simulink model "Part3_simulazione"  (R2024b)
settings: Solver=ode4  StartTime=0.0  StopTime=T_SIM  FixedStep=T_s  RelTol=1e-3
values from neighbouring files (symbols this model uses):
  D = diag([0.001, 0.001, 0.0175/6, 0.0175/6, 0.0175/6, 0.0175/6*T_s, 0.0175/6*T_s].^2)    [P2_script.m]    (also in P3_script_usare_dati_veri.m; Parte2_corretto.m)
  d = 0.165    [P1_script.m]    (also in P1_script_vers2.m; P2_script.m; P3_script.m; P3_script_usare_dati_veri.m = 0.18428)
  d_id = d_cal_hat    [P2_script.m]    (also in P3_script_usare_dati_veri.m = 0.18428; Parte2_corretto.m)
  H_enc = [0, 0, 0, 1, 0, 0, 0 ... (first row only)    [P2_script.m]    (also in P3_script_usare_dati_veri.m; Parte2_corretto.m)
  H_gyro = [0, 0, 0, 0, 0, -r_id/d_id, r_id/d_id]    [P2_script.m]    (also in P3_script_usare_dati_veri.m; Parte2_corretto.m)
  H_motion_cap = [1, 0, 0, 0, 0, 0, 0 ... (first row only)    [P2_script.m]    (also in P3_script_usare_dati_veri.m; Parte2_corretto.m)
  omega_max = 10    [P1_script.m]    (also in P1_script_vers2.m; P2_script.m; P3_script.m; P3_script_usare_dati_veri.m)
  P_INIT_EKF = diag([0.001, 0.001, 0.0175/6, 0.0175/6, 0.0175/6, 0.0175/6*T_s, 0.0175/6*T_s].^2)    [P2_script.m]    (also in P3_script_usare_dati_veri.m; Parte2_corretto.m)
  p_loss = p_loss_values(3)    [P2_script.m]    (also in P3_script_usare_dati_veri.m = p_loss_values(i); Parte2_corretto.m = p_loss_values(2))
  PHI_INIT = [0;0]    [P1_script.m]    (also in P1_script_vers2.m; P2_script.m; P3_script_usare_dati_veri.m; Parte2_corretto.m)
  Q_INIT = [0; 0; atan2((R*omega_trj), (2*R*omega_trj))]    [P1_script.m]    (also in P1_script_vers2.m = q(:,1); P2_script.m = q_motion_capture_cal(1,:)'; P3_script_usare_dati_veri.m = q_motion_capture(1,:)'; Parte2_corretto.m = q_motion_capture_cal(1,:)')
  Q_INIT_LOC = Q_INIT    [P1_script.m]    (also in P1_script_vers2.m; P2_script.m; P3_script_usare_dati_veri.m = Q_INIT + [0.2; 0.2; deg2rad(15)]; Parte2_corretto.m)
  r = 0.03    [P1_script.m]    (also in P1_script_vers2.m; P2_script.m; P3_script.m; P3_script_usare_dati_veri.m = 0.03316)
  R_3 = diag(([var_motion_capture, var_motion_capture, var_motion_capture,               ENCODER_QUANTIZATION/6, ENCODER_QUANTIZATION/6, var_IMU]).^2)    [P2_script.m]    (also in P3_script_usare_dati_veri.m; Parte2_corretto.m)
  r_id = r_cal_hat    [P2_script.m]    (also in P3_script_usare_dati_veri.m = 0.03316; Parte2_corretto.m)
  T_s = 0.04    [P1_script.m]    (also in P1_script_vers2.m; P2_script.m; P3_script.m; P3_script_usare_dati_veri.m)
  Ts = 1e-2    (= 0.01)    [collaudo.m]
  Z_INIT_EKF = [Q_INIT; 0; 0; 0; 0]    [P1_script.m]    (also in P1_script_vers2.m; P2_script.m; P3_script_usare_dati_veri.m = [Q_INIT_LOC; 0; 0; 0; 0]; Parte2_corretto.m = [Q_INIT_LOC; 0; 0; 0; 0])
undefined symbols (not defined in the file or in its folder): X, Y
libraries: robotlib x5
settings Model: Creator=tomailoren  LastModifiedBy=loren
settings OptimizationCC: DefaultParameterBehavior=Inlined  EnhancedBackFolding=on  PassReuseOutputArgsAs=Individual arguments  ZeroExternalMemoryAtStartup=off  ZeroInternalMemoryAtStartup=off  MaxStackSize=64  OptimizeBlockOrder=speed  DifferentSizesBufferReuse=on  OptimizationCustomize=off  EfficientTunableParamExpr=on
settings DebuggingCC: ParameterTunabilityLossMsg=error
settings HardwareCC: ProdBitPerPointer=32  ProdBitPerSizeT=32  ProdBitPerPtrDiffT=32  ProdLargestAtomicFloat=None  ProdIntDivRoundTo=Undefined  ProdEndianess=Unspecified  ProdWordSize=32  ProdHWDeviceType=Generic->Unspecified (assume 32-bit Generic)
settings SFSimCC: MATLABDynamicMemAlloc=off
settings RTWCC: Description=Embedded Coder  SystemTargetFile=ert.tlc  HardwareBoard=Robot Operating System (ROS)  TLCOptions="-aInlineSetEventsForThisBaseRateFcn=TLC_FALSE -aSuppressMultiTaskScheduler=TLC_FALSE  -aRateBasedStepFcn=0"  TemplateMakefile=ert_default_tmf  Toolchain=Catkin  TargetLang=C++
settings CodeAppCC: ForceParamTrailComments=on  IgnoreCustomStorageClasses=off  OperatorAnnotations=on  SimulinkDataObjDesc=on  SFDataObjDesc=on  InsertBlockDesc=on

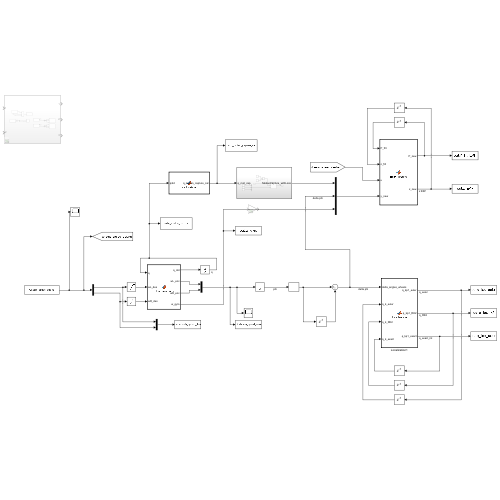
[thumbnail: Simulink's stored preview of the top-level diagram]
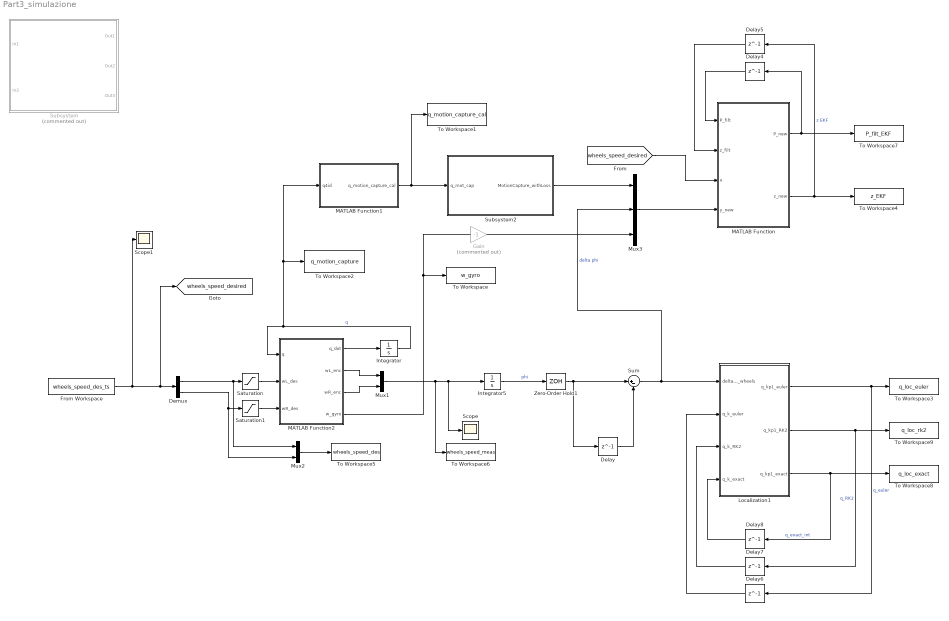
== system Part3_simulazione ==
  Delay : Delay  DelayLength=1  InitialCondition=[0;0]  SampleTime=T_s
  Delay4 : Delay  DelayLength=1  InitialCondition=P_INIT_EKF  SampleTime=T_s
  Delay5 : Delay  DelayLength=1  InitialCondition=Z_INIT_EKF  SampleTime=T_s
  Delay6 : Delay  DelayLength=1  InitialCondition=Q_INIT_LOC
  Delay7 : Delay  DelayLength=1  InitialCondition=Q_INIT_LOC
  Delay8 : Delay  DelayLength=1  InitialCondition=Q_INIT_LOC
  Demux : Demux  Outputs=2
  From Workspace : FromWorkspace  VariableName=wheels_speed_des_ts
  Gain : Gain  Commented=on  Gain=-1
  Integrator : Integrator  InitialCondition=Q_INIT
  Integrator5 : Integrator  InitialCondition=PHI_INIT
  Localization1 : MATLAB Function  TreatAsAtomicUnit=on
  MATLAB Function : MATLAB Function  TreatAsAtomicUnit=on
  MATLAB Function1 : MATLAB Function  TreatAsAtomicUnit=on
  MATLAB Function2 : MATLAB Function  TreatAsAtomicUnit=on
  Mux1 : Mux  Inputs=2
  Mux2 : Mux  Inputs=2
  Mux3 : Mux  Inputs=3
  Saturation : Saturate  UpperLimit=omega_max  LowerLimit=-omega_max
  Saturation1 : Saturate  UpperLimit=omega_max  LowerLimit=-omega_max
  Scope : Scope
  Scope1 : Scope
  Subsystem : Subsystem  Commented=on
  Subsystem2 : Subsystem
  Sum : Sum  Inputs=|+-
  To Workspace : ToWorkspace  VariableName=w_gyro  SaveFormat=Structure With Time  SampleTime=-1
  To Workspace1 : ToWorkspace  VariableName=q_motion_capture_cal  SaveFormat=Structure With Time  SampleTime=-1
  To Workspace2 : ToWorkspace  VariableName=q_motion_capture  SaveFormat=Structure With Time  SampleTime=-1
  To Workspace3 : ToWorkspace  VariableName=q_loc_euler  SaveFormat=Structure With Time  SampleTime=-1
  To Workspace4 : ToWorkspace  VariableName=z_EKF  SaveFormat=Structure With Time  SampleTime=-1
  To Workspace5 : ToWorkspace  VariableName=wheels_speed_des  SaveFormat=Structure With Time  SampleTime=-1
  To Workspace6 : ToWorkspace  VariableName=wheels_speed_meas  SaveFormat=Structure With Time  SampleTime=-1
  To Workspace7 : ToWorkspace  VariableName=P_filt_EKF  SaveFormat=Structure With Time  SampleTime=-1
  To Workspace8 : ToWorkspace  VariableName=q_loc_exact  SaveFormat=Structure With Time  SampleTime=-1
  To Workspace9 : ToWorkspace  VariableName=q_loc_rk2  SaveFormat=Structure With Time  SampleTime=-1
  Zero-Order Hold1 : ZeroOrderHold  SampleTime=T_s
  tag scope: wheels_speed_desired=global
  wires:
  Mux1/1 -> Scope/1, Integrator5/1, To Workspace6/1
  Zero-Order Hold1/1 -> Sum/1, Delay/1
  Delay/1 -> Sum/2
  Integrator5/1 -> Zero-Order Hold1/1  "phi"
  MATLAB Function2/2(wL_enc) -> Mux1/1
  MATLAB Function2/3(wR_enc) -> Mux1/2
  Demux/1 -> Mux2/1, Saturation/1
  Saturation/1 -> MATLAB Function2/2(wL_des)
  Demux/2 -> Mux2/2, Saturation1/1
  Saturation1/1 -> MATLAB Function2/3(wR_des)
  Mux2/1 -> To Workspace5/1
  From Workspace/1 -> Scope1/1, [wheels_speed_desired], Demux/1
  Delay5/1 -> MATLAB Function/2(z_filt)
  MATLAB Function/2(z_new) -> Delay5/1, To Workspace4/1  "z EKF"
  Delay4/1 -> MATLAB Function/1(P_filt)
  MATLAB Function/1(P_new) -> Delay4/1, To Workspace7/1
  Localization1/3(q_kp1_exact) -> To Workspace8/1, Delay8/1  "q_exact_int"
  Localization1/1(q_kp1_euler) -> To Workspace3/1, Delay6/1  "q_euler"
  Delay6/1 -> Localization1/2(q_k_euler)
  Localization1/2(q_kp1_RK2) -> To Workspace9/1, Delay7/1  "q_RK2"
  Delay8/1 -> Localization1/4(q_k_exact)
  Delay7/1 -> Localization1/3(q_k_RK2)
  Subsystem2/1(MotionCapture_withLoss) -> Mux3/1
  Sum/1 -> Mux3/2, Localization1/1(delta_angles_wheels)  "delta phi"
  MATLAB Function2/4(w_gyro) -> To Workspace/1, Mux3/3
  Mux3/1 -> MATLAB Function/4(y_new)
  MATLAB Function1/1(q_motion_capture_cal) -> To Workspace1/1, Subsystem2/1(q_mot_cap)
  [wheels_speed_desired] -> MATLAB Function/3(u)
  MATLAB Function2/1(q_dot) -> Integrator/1
  Integrator/1 -> MATLAB Function1/1(q4id), To Workspace2/1, MATLAB Function2/1(q)  "q"

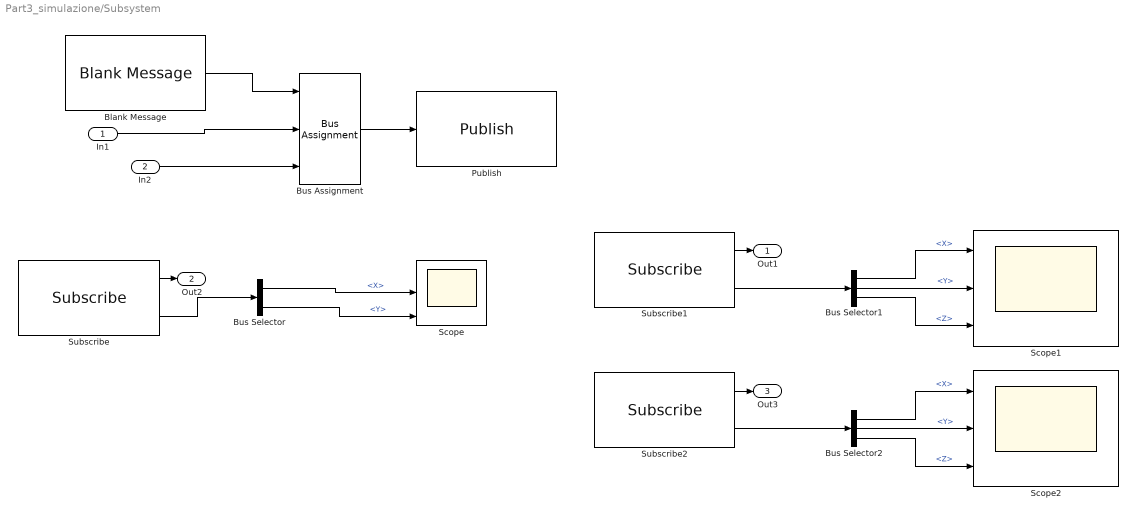
== system Part3_simulazione/Subsystem ==
  In1 : Inport
  In2 : Inport  Port=2
  Blank Message : robotlib/Blank Message  messageClass=Message  entityType=geometry_msgs/Vector3  messageType=geometry_msgs/Vector3  SampleTime=Ts  legacyBusStruct=off
  Bus Assignment : BusAssignment  AssignedSignals=X,Y
  Bus Selector : BusSelector  OutputSignals=X,Y
  Bus Selector1 : BusSelector  OutputSignals=X,Y,Z
  Bus Selector2 : BusSelector  OutputSignals=X,Y,Z
  Publish : robotlib/Publish  topicSource=Select from ROS network  topic=/turtlebot_01/cmd_wheels  messageType=geometry_msgs/Vector3  legacyBusStruct=off  messageQueueLength=1
  Scope : Scope  NumInputPorts=3
  Scope1 : Scope  NumInputPorts=3
  Scope2 : Scope  NumInputPorts=3
  Subscribe : robotlib/Subscribe  topicSource=Select from ROS network  topic=/turtlebot_01/wheelSpeeds  messageType=geometry_msgs/Vector3  SampleTime=Ts  legacyBusStruct=off  messageQueueLength=1
  Subscribe1 : robotlib/Subscribe  topicSource=Select from ROS network  topic=/turtlebot_01/gyroscope  messageType=geometry_msgs/Vector3  SampleTime=Ts  legacyBusStruct=off  messageQueueLength=1
  Subscribe2 : robotlib/Subscribe  topicSource=Select from ROS network  topic=/turtlebot_01/accelerometer  messageType=geometry_msgs/Vector3  SampleTime=Ts  legacyBusStruct=off  messageQueueLength=1
  Out1 : Outport
  Out2 : Outport  Port=2
  Out3 : Outport  Port=3
  wires:
  Bus Selector1/2 -> Scope1/2  "<Y>"
  Subscribe/2 -> Bus Selector/1
  Bus Selector2/1 -> Scope2/1  "<X>"
  Bus Selector1/3 -> Scope1/3  "<Z>"
  Bus Selector2/2 -> Scope2/2  "<Y>"
  Subscribe1/1 -> Out1/1
  Bus Assignment/1 -> Publish/1
  Bus Selector1/1 -> Scope1/1  "<X>"
  Bus Selector/1 -> Scope/2  "<X>"
  In2/1 -> Bus Assignment/3
  Subscribe1/2 -> Bus Selector1/1
  Subscribe2/2 -> Bus Selector2/1
  Blank Message/1 -> Bus Assignment/1
  Bus Selector/2 -> Scope/3  "<Y>"
  Bus Selector2/3 -> Scope2/3  "<Z>"
  In1/1 -> Bus Assignment/2
  Subscribe2/1 -> Out3/1
  Subscribe/1 -> Out2/1

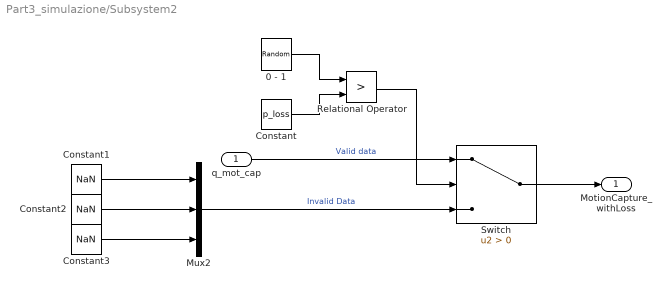
== system Part3_simulazione/Subsystem2 ==
  q_mot_cap : Inport
  0 - 1 : UniformRandomNumber  Minimum=0  SampleTime=T_s
  Constant : Constant  Value=p_loss
  Constant1 : Constant  Value=NaN
  Constant2 : Constant  Value=NaN
  Constant3 : Constant  Value=NaN
  Mux2 : Mux  Inputs=3
  Relational Operator : RelationalOperator  Operator=>  OutDataTypeStr=boolean  RndMeth=Simplest  InputSameDT=off
  Switch : Switch  Criteria=u2 > Threshold  SaturateOnIntegerOverflow=off  InputSameDT=off
  MotionCapture_withLoss : Outport
  wires:
  0 - 1/1 -> Relational Operator/1
  Constant/1 -> Relational Operator/2
  Switch/1 -> MotionCapture_withLoss/1
  Relational Operator/1 -> Switch/2
  Constant2/1 -> Mux2/2
  Mux2/1 -> Switch/3  "Invalid Data"
  Constant1/1 -> Mux2/1
  q_mot_cap/1 -> Switch/1  "Valid data"
  Constant3/1 -> Mux2/3

== matlab function Part3_simulazione/Localization1 ==
  data: delta_angles_wheels input; q_k_euler input; q_k_RK2 input; q_k_exact input; r_id parameter; d_id parameter; q_kp1_euler output; T_s parameter; q_kp1_RK2 output; q_kp1_exact output
function [q_kp1_euler, q_kp1_RK2, q_kp1_exact] = localization(delta_angles_wheels, q_k_euler, q_k_RK2, q_k_exact, r_id, d_id, T_s)

    r = r_id;
    d = d_id;

    % extraction data
    delta_phi_L = delta_angles_wheels(1);
    delta_phi_R = delta_angles_wheels(2);

    x_k_euler = q_k_euler(1); 
    y_k_euler = q_k_euler(2); 
    theta_k_euler = q_k_euler(3);
    
    x_k_RK2 = q_k_RK2(1); 
    y_k_RK2 = q_k_RK2(2); 
    theta_k_RK2 = q_k_RK2(3);

    x_k_exact = q_k_exact(1);
    y_k_exact = q_k_exact(2); 
    theta_k_exact = q_k_exact(3);


    % velocities estimate
    v_k = r / (2*T_s) * (delta_phi_R + delta_phi_L);
    w_k = r / (d*T_s) * (delta_phi_R - delta_phi_L);
    
    % Euler integration
    x_kp1_euler = x_k_euler + v_k * T_s * cos(theta_k_euler);
    y_kp1_euler = y_k_euler + v_k * T_s * sin(theta_k_euler);
    theta_kp1_euler = theta_k_euler + w_k * T_s;
    
    q_kp1_euler = [x_kp1_euler; y_kp1_euler; theta_kp1_euler];
    
    % RK2 Integration
    x_kp1_RK2 = x_k_RK2 + v_k * T_s * cos(theta_k_RK2 + (w_k * T_s)/2);
    y_kp1_RK2 = y_k_RK2 + v_k * T_s * sin(theta_k_RK2 + (w_k * T_s)/2);
    theta_kp1_RK2 = theta_k_RK2 + w_k * T_s;
    
    q_kp1_RK2 = [x_kp1_RK2; y_kp1_RK2; theta_kp1_RK2];
    
    % Exact Integration
    if abs(w_k) < 1e-4
        % use RK2 approximation to avoid division by zero when w_k is near 0
        x_kp1_exact = x_k_exact + v_k * T_s * cos(theta_k_exact + (w_k * T_s)/2);
        y_kp1_exact = y_k_exact + v_k * T_s * sin(theta_k_exact + (w_k * T_s)/2);
    else
        % Exact formulas
        x_kp1_exact = x_k_exact + (v_k / w_k) * (sin(theta_k_exact + w_k * T_s) - sin(theta_k_exact));
        y_kp1_exact = y_k_exact - (v_k / w_k) * (cos(theta_k_exact + w_k * T_s) - cos(theta_k_exact));
    end
    theta_kp1_exact = theta_k_exact + w_k * T_s;
    
    q_kp1_exact = [x_kp1_exact; y_kp1_exact; theta_kp1_exact];
    
end

== matlab function Part3_simulazione/MATLAB Function1 ==
  data: q4id input; q_motion_capture_cal output
function q_motion_capture_cal = calibration(q4id)

x_off_cal = -0.00434;
y_off_cal = 0.00361;
theta_off = -0.02331;


theta_cal = q4id(3) - theta_off;
x_cal = q4id(1) - (x_off_cal * cos(theta_cal) - y_off_cal * sin(theta_cal));
y_cal = q4id(2) - (x_off_cal * sin(theta_cal) + y_off_cal * cos(theta_cal));


q_motion_capture_cal = [x_cal; y_cal; theta_cal];

== matlab function Part3_simulazione/MATLAB Function2 ==
  data: q input; q_dot output; wL_des input; wR_des input; wL_enc output; wR_enc output; w_gyro output; r parameter; d parameter; T_s parameter
function [q_dot, wL_enc, wR_enc, w_gyro] = robot_simulator(q, wL_des, wR_des, r, d, T_s)
    
    wL_enc = wL_des;
    wR_enc = wR_des;
      
    v = (r/2) * (wR_des + wL_des);
    omega = (r/d) * (wR_des - wL_des);
    
    w_gyro = -omega;
    
    q_dot= zeros(3,1);
    
    q_dot(1) = v*cos(q(3));
    q_dot(2) = v*sin(q(3));
    q_dot(3) = omega;
    
end

== matlab function Part3_simulazione/MATLAB Function ==
  data: P_filt input; P_new output; z_filt input; z_new output; u input; y_new input; D parameter; T_s parameter; r_id parameter; d_id parameter; H_enc parameter; H_gyro parameter; H_motion_cap parameter; R_3 parameter
function [P_new, z_new] = EKF_filtering(P_filt, z_filt, u, y_new, D, T_s, r_id, d_id, H_enc, H_gyro, H_motion_cap, R_3)

    % Def state z_filt: [xk , yk , thetak , delta_phi_L_km1 , delta_phi_R_km1 , wLk , wRk ]

    r = r_id;
    d = d_id;
        
    % Extraction variables
    x_k = z_filt(1);
    y_k = z_filt(2);
    theta_k = z_filt(3);
    delta_phi_L_km1 = z_filt(4);
    delta_phi_R_km1 = z_filt(5); 
    wL_k = z_filt(6);               % estimate wheels velocities
    wR_k = z_filt(7);
    
    uL_k = u(1);                    % actual wheels velocities (from command input v,w)
    uR_k = u(2);

    % ----------------------

    % PREDICT STEP
    v_k = (r/2) * (wL_k + wR_k);
    omega_k = (r/d) * (wR_k - wL_k);
    theta_mean = theta_k + (omega_k * T_s) / 2;
        
    % State Prediction (approximation with RK2)
    x_kp1 = x_k + v_k * T_s * cos(theta_mean);
    y_kp1 = y_k + v_k * T_s * sin(theta_mean);
    theta_kp1 = theta_k + omega_k * T_s;
    
    delta_phi_L_k = wL_k * T_s;
    delta_phi_R_k = wR_k * T_s;
    
    wL_kp1 = uL_k; 
    wR_kp1 = uR_k;
    
    z_hat = [x_kp1; y_kp1; theta_kp1; delta_phi_L_k; delta_phi_R_k; wL_kp1; wR_kp1];
    
    % F derivation
    F = zeros(7,7);
    
    F(1,1) = 1;
    F(1, 3) = -T_s * v_k * sin(theta_mean);
    F(1, 6) = (T_s * r / 2) * cos(theta_mean) - v_k * T_s * sin(theta_mean) * (-T_s * r / (2 * d));
    F(1, 7) = (T_s * r / 2) * cos(theta_mean) - v_k * T_s * sin(theta_mean) * (T_s * r / (2 * d));
    
    F(2,2) = 1;
    F(2, 3) = v_k * T_s * cos(theta_mean);
    F(2, 6) = (T_s * r / 2) * sin(theta_mean) + v_k * T_s * cos(theta_mean) * (-T_s * r / (2 * d));
    F(2, 7) = (T_s * r / 2) * sin(theta_mean) + v_k * T_s * cos(theta_mean) * (T_s * r / (2 * d));

    F(3,3) = 1;
    F(3, 6) = -T_s * r / d;
    F(3, 7) = T_s * r / d;

    F(4, 6) = T_s;
    F(5, 7) = T_s;
    
    % Covariance Prediction
    P_hat = F * P_filt * F' + D;
    
    % ----------------------

    % UPDATE STEP
    % H and R will depend on the measurement data y_new and Test_case

    % enc_values (delta_phi)
    % IMU_values (w_gyro)
    % Motion_capture (state q)

    % y_new = [x; y; theta; delta_phi_L; delta_phi_R; omega_gyro]

    %% OBSERVATION MATRIX H ALWAYS FULL (6X7) AND ALSO Y_NEW (6X1) 
    H_full = [H_motion_cap; H_enc; H_gyro];
    y_meas = y_new; 
    
    % Usiamo la R_3 (6x6) come base
    R_current = R_3;
    INFINITY_VAR = 1e9; % Incertezza "infinita" per spegnere il Kalman Gain
    
    % TEST 3: Tutti attivi, perdita pacchetto Mocap dinamica
    if any(isnan(y_new(1:3)))
        y_meas(1:3) = 0; % Mocap perso -> forziamo a zero
        R_current(1,1) = INFINITY_VAR; R_current(2,2) = INFINITY_VAR; R_current(3,3) = INFINITY_VAR;
    end

    
    % Innovation e_pred
    y_hat = H_full * z_hat;
    e_kp1 = y_meas - y_hat;
    
    % Kalman Gain K_pred
    K = P_hat * H_full' / (H_full * P_hat * H_full' + R_current);   
    
    % State and Covariance Update
    z_new = z_hat + K * e_kp1;
    P_new = P_hat - K * H_full * P_hat;


end
